simulink model "full_loop"  (R2020a)
settings: Solver=FixedStepAuto  StartTime=0.0  StopTime=inf  FixedStep=.005  RelTol=1e-3
undefined symbols (not defined in the file or in its folder): cf, gazeboStep
libraries: robotlib x2, sharedutil x1
settings Model: EnablePacing=on  Creator=Lamarre  LastModifiedBy=lamarre

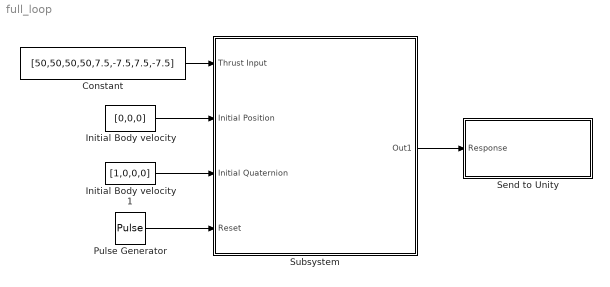
== system full_loop ==
  Constant : Constant  Value=[50,50,50,50,7.5,-7.5,7.5,-7.5]
  "Initial Body velocity " : Constant  Value=[0,0,0]
  Initial Body velocity 1 : Constant  Value=[1,0,0,0]
  Pulse Generator : DiscretePulseGenerator  PulseType=Time based  Period=10  PulseWidth=0.05
  Send to Unity : Subsystem  InitFcn=|
      | cf = ConfigAUV8();
      | 
      | % Parametres Messages ROS
      |     Duration = 229;
      |     gazeboStep=1/50;
      |     telemetryStep=1/30;
      |     referenceFrame = cf.referenceFrame;
      |     modelName = cf.modelName;
  Subsystem : Subsystem
  wires:
  Constant/1 -> Subsystem/1(Thrust Input)
  Subsystem/1(Out1) -> Send to Unity/1(Response)
  "Initial Body velocity "/1 -> Subsystem/2(Initial Position)
  Initial Body velocity 1/1 -> Subsystem/3(Initial Quaternion)
  Pulse Generator/1 -> Subsystem/4(Reset)

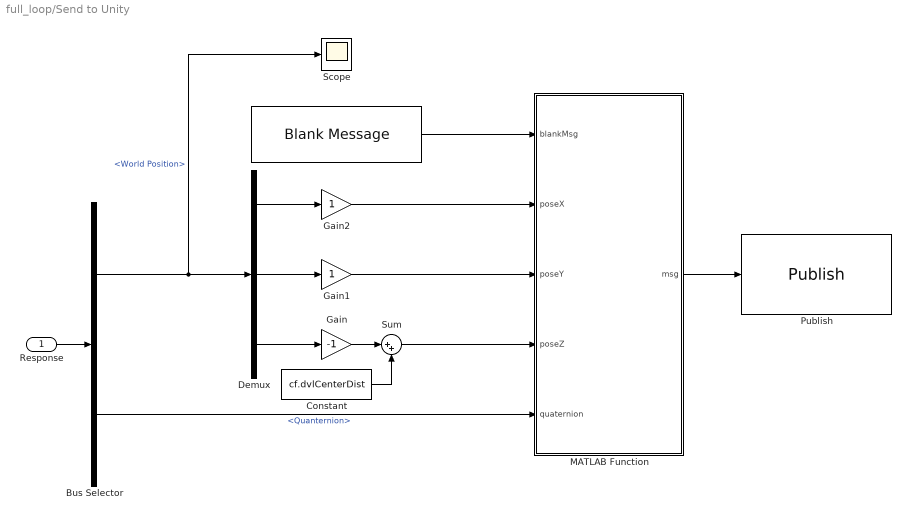
== system full_loop/Send to Unity ==
  Response : Inport
  "   " : robotlib/Blank Message  messageClass=Message  entityType=auv_package/PosRot  messageType=auv_package/PosRot  SampleTime=1/50
  Bus Selector : BusSelector  OutputSignals=World Position,Quanternion
  Constant : Constant  Value=cf.dvlCenterDist
  Demux : Demux  Outputs=3
  Gain : Gain  Gain=-1
  Gain1 : Gain
  Gain2 : Gain
  MATLAB Function : MATLAB Function  TreatAsAtomicUnit=on  SystemSampleTime=gazeboStep
  Publish : robotlib/Publish  topicSource=Specify your own  topic=/pos_rot  messageType=auv_package/PosRot  messageQueueLength=1
      link override SinkBlock: ROSTopic=/gazebo/set_model_state  ROSMessageType=gazebo_msgs/ModelState  SLBusName=SL_Bus_plant_gazebo_msgs_ModelState  ModelName=plant  BlockId=Pub_plant_206
  Scope : Scope
  Sum : Sum  Inputs=|++
  wires:
  Bus Selector/1 -> Scope/1, Demux/1  "<World Position>"
  Demux/1 -> Gain2/1
  Demux/2 -> Gain1/1
  Demux/3 -> Gain/1
  "   "/1 -> MATLAB Function/1(blankMsg)
  Gain1/1 -> MATLAB Function/3(poseY)
  Bus Selector/2 -> MATLAB Function/5(quaternion)  "<Quanternion>"
  Gain2/1 -> MATLAB Function/2(poseX)
  MATLAB Function/1(msg) -> Publish/1
  Response/1 -> Bus Selector/1
  Gain/1 -> Sum/1
  Sum/1 -> MATLAB Function/4(poseZ)
  Constant/1 -> Sum/2

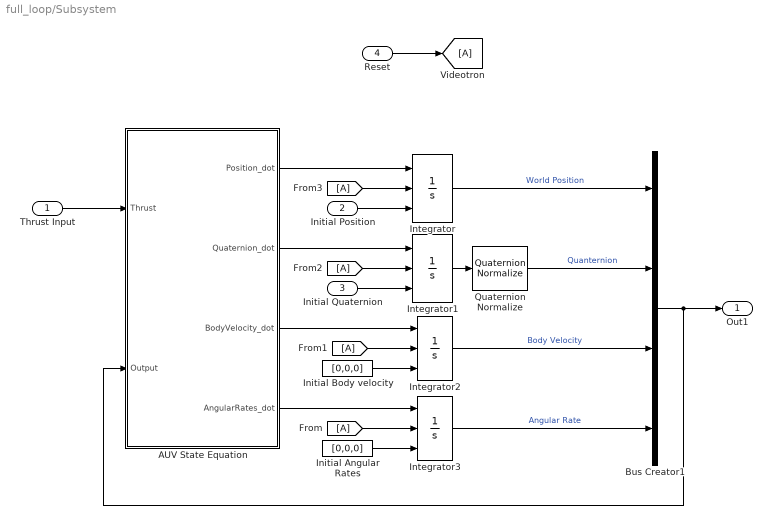
== system full_loop/Subsystem ==
  Thrust Input : Inport
  Initial Position : Inport  Port=2
  Initial Quaternion : Inport  Port=3
  Reset : Inport  Port=4
  AUV State Equation : MATLAB Function  TreatAsAtomicUnit=on  SystemSampleTime=.005
  Bus Creator1 : BusCreator  Inputs=4
  Initial Angular Rates : Constant  Value=[0,0,0]
  "Initial Body velocity " : Constant  Value=[0,0,0]
  Integrator : Integrator  ExternalReset=rising  InitialConditionSource=external  InitialCondition=[0,0,1]
  Integrator1 : Integrator  ExternalReset=rising  InitialConditionSource=external  InitialCondition=[1,0,0,0]
  Integrator2 : Integrator  ExternalReset=rising  InitialConditionSource=external  InitialCondition=[0,0,0]
  Integrator3 : Integrator  ExternalReset=rising  InitialConditionSource=external  InitialCondition=[0,0,0]
  Quaternion Normalize : sharedutil/Quaternion Normalize  aMode=aMode
      settings: SourceProductBaseCode=AE,PW,MT,VE,VP
  Out1 : Outport
  wires:
  "Initial Body velocity "/1 -> Integrator2/3
  Integrator1/1 -> Quaternion Normalize/1
  AUV State Equation/2(Quaternion_dot) -> Integrator1/1
  Integrator/1 -> Bus Creator1/1  "World Position"
  Integrator2/1 -> Bus Creator1/3  "Body Velocity"
  AUV State Equation/1(Position_dot) -> Integrator/1
  Initial Angular Rates/1 -> Integrator3/3
  Bus Creator1/1 -> Out1/1, AUV State Equation/2(Output)
  Thrust Input/1 -> AUV State Equation/1(Thrust)
  AUV State Equation/4(AngularRates_dot) -> Integrator3/1
  Quaternion Normalize/1 -> Bus Creator1/2  "Quanternion"
  Integrator3/1 -> Bus Creator1/4  "Angular Rate"
  Initial Quaternion/1 -> Integrator1/3
  AUV State Equation/3(BodyVelocity_dot) -> Integrator2/1
  [A] -> Integrator3/2
  [A] -> Integrator2/2
  [A] -> Integrator1/2
  [A] -> Integrator/2
  Initial Position/1 -> Integrator/3
  Reset/1 -> [A]

== matlab function full_loop/Subsystem/AUV State Equation ==
  data: Thrust input; Output input; Position_dot output size=3; Quaternion_dot output size=4; BodyVelocity_dot output size=3; AngularRates_dot output size=3
function [Position_dot,Quaternion_dot,BodyVelocity_dot, AngularRates_dot] = AUVStateEquation(Thrust,Output)

Dynamics=AUVFossenSimFcn(Output,Thrust);

Position_dot=Dynamics(1:3);
Quaternion_dot = Dynamics(4:7);
BodyVelocity_dot= Dynamics(8:10);
AngularRates_dot = Dynamics(11:13);

== matlab function full_loop/Send to Unity/MATLAB Function ==
  data: blankMsg input; poseX input; poseY input; poseZ input; msg output SL_Bus_full_loop_auv_package_PosRot; quaternion input
function msg = assignUnityPoseRotInput(blankMsg, poseX, poseY, poseZ, quaternion)
% assignStringInput - Assign a string in a ROS message to specified input string
%
% MSG = assignStringInput(blankMsg, STR) assigns the input string, STR, to
%  a string field in the ROS message, blankMsg, and outputs the updated
%  ROS message.
%
%  Inputs
%    blankMsg: A bus for a 'std_msgs/String' message. This is 
%        used to initialize the output.
%    str: An array of uint8 that will be assigned to the 'Data' field
%        in blankMsg. The entire array is assumed to be a valid sequence of
%        character ASCII values.
% 
%  Outputs:
%    msg: A bus for a 'std_msgs/String' message, with the 'Data'
%        field set to a string.

%   Copyright 2015 The MathWorks, Inc.
%#codegen

% Note: The datatype of 'msg' has been explicitly set to the appropriate 
% Simulink bus type ("Bus: SL_Bus_robotROSMessageUsageExample_std_msgs_String"). 
%
% If the model name is changed, the datatype needs to be changed as well:
%   1) Click "Edit Data" in the Editor toolstrip to open "Ports and Data Manager"
%   2) Select "msg". From the "Type" dropdown, select "--- Refresh data types ---"
%   3) Set datatype to "Bus: SL_Bus_<modelname>_std_msgs_String"
   
msg = blankMsg;


msg.PosX = cast(poseX,'single');
msg.PosY = cast(poseY,'single');
msg.PosZ = cast(poseZ,'single');

msg.RotW = cast(quaternion(1),'single');
msg.RotX = cast(quaternion(2),'single');
msg.RotY = cast(quaternion(3),'single');
msg.RotZ = cast(quaternion(4),'single');
